simulink model "Spunto2"  (R2022a)
settings: Solver=VariableStepAuto  StartTime=0.0  StopTime=30  RelTol=1e-3
settings Model: Creator=bryan  LastModifiedBy=bryan

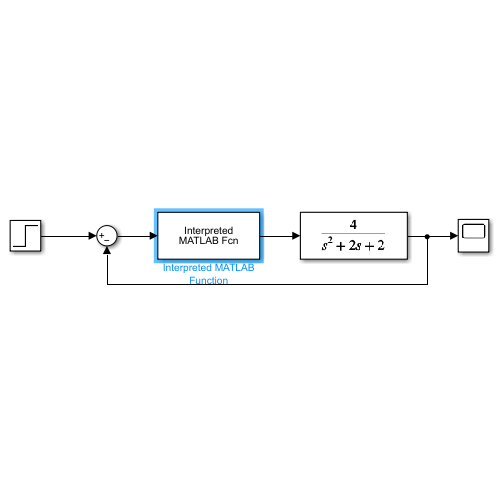
[thumbnail: Simulink's stored preview of the top-level diagram]
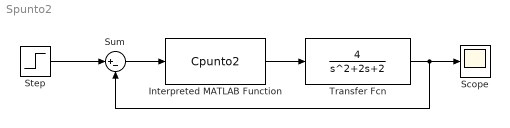
== system Spunto2 ==
  Interpreted MATLAB Function : MATLABFcn  MATLABFcn=Cpunto2
  Scope : Scope
  Step : Step  SampleTime=0
  Sum : Sum  Inputs=|+-
  Transfer Fcn : TransferFcn  Numerator=[4]  Denominator=[1 2 2]
  wires:
  Step/1 -> Sum/1
  Sum/1 -> Interpreted MATLAB Function/1
  Interpreted MATLAB Function/1 -> Transfer Fcn/1
  Transfer Fcn/1 -> Scope/1, Sum/2
